simulink model "sampleModel1937"  (R2023a)
settings: Solver=VariableStepAuto  StartTime=0.0  StopTime=10.0  RelTol=1e-3
libraries: hdlsllib x6, simulink x2
settings Model: Creator=user1  LastModifiedBy=user1

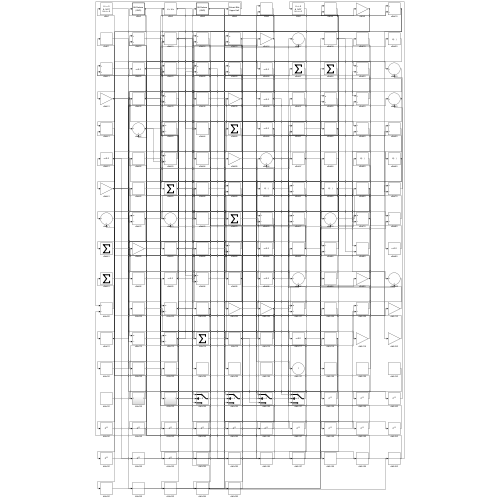
[thumbnail: Simulink's stored preview of the top-level diagram]
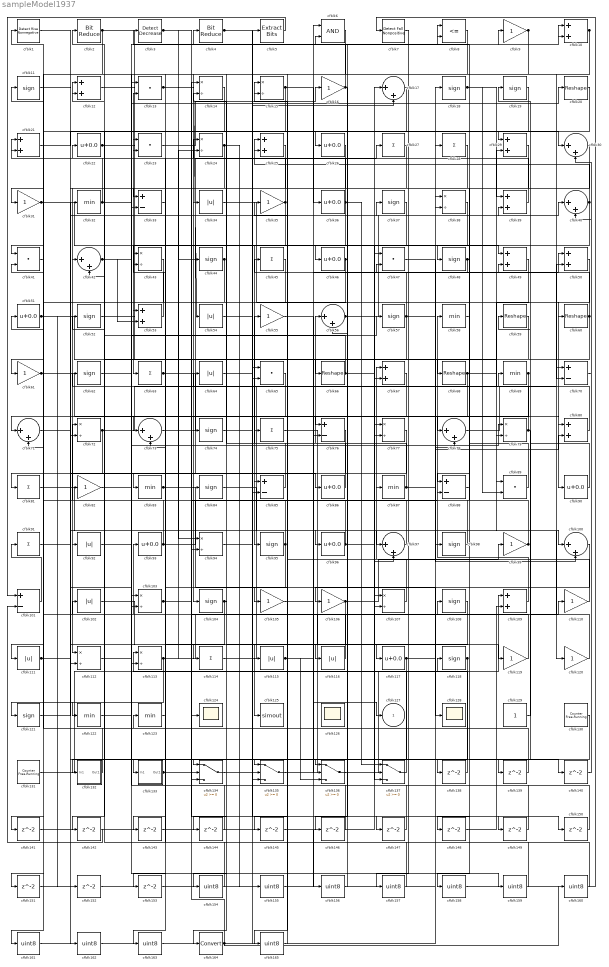
== system sampleModel1937 ==
  cfblk1 : hdlsllib/Logic and Bit Operations/Detect Rise Nonnegative  vinit=0  OutDataTypeStr=boolean
  cfblk{10,12,21,25,29,39,49..50,53,67,80,109} (12 alike) : Sum
  cfblk{17,30,40,42,56,71,73,78,97,100} (10 alike) : Sum  Inputs=|++
  cfblk{33,70,76,85,88,101} (6 alike) : Sum  Inputs=+-
  cfblk{34,54,64,92,102,111,115..116} (8 alike) : Abs  SaturateOnIntegerOverflow=off
  cfblk{14..15,24,38,43,72,77,79,94,103,107,112..113} (13 alike) : Product  Inputs=*/  RndMeth=Zero  SaturateOnIntegerOverflow=on
  cfblk{11,18..19,37,44,48,52,57,62,74,84,95,98,104,108,118,121} (17 alike) : Signum
  cfblk{9,16,31,35,55,61,82,99,105..106,110,119..120} (13 alike) : Gain
  cfblk{27..28,45,63,75,81,91,114} (8 alike) : Sum  Inputs=+
  cfblk{22,26,36,46,51,86,90,93,96,117} (10 alike) : Bias  Bias=0.0  SaturateOnIntegerOverflow=off
  cfblk{32,58,69,83,87,122..123} (7 alike) : MinMax
  cfblk124 : Scope
  cfblk125 : ToWorkspace  VariableName=simout  SaveFormat=Timeseries  SampleTime=-1
  cfblk126 : Scope
      settings: Floating=on
  cfblk128 : Scope
  cfblk129 : Constant  SampleTime=-1
  cfblk{13,23,41,47,65,89} (6 alike) : DotProduct  OutDataTypeStr=Inherit: Inherit via internal rule
  cfblk130 : hdlsllib/Sources/Counter Free-Running  NumBits=16  tsamp=-1
  cfblk131 : hdlsllib/Sources/Counter Free-Running  NumBits=16  tsamp=-1
  cfblk132 : Subsystem
      settings: LibrarySourceBlock=|
      | hdlsllib/Ports &
      | Subsystems/Subsystem
  cfblk133 : Subsystem
      settings: LibrarySourceBlock=|
      | hdlsllib/Ports &
      | Subsystems/Subsystem
  cfblk{134..137} (4 alike) : Switch  SaturateOnIntegerOverflow=off  InputSameDT=off
  cfblk{138..153} (16 alike) : Delay  SampleTime=1
  cfblk{154..163,165} (11 alike) : DataTypeConversion  OutDataTypeStr=uint8  SaturateOnIntegerOverflow=off  RndMeth=Floor
  cfblk164 : DataTypeConversion  SaturateOnIntegerOverflow=off  RndMeth=Floor
  cfblk2 : hdlsllib/Logic and Bit Operations/Bit Reduce  mode=AND
  cfblk{20,59..60,66,68} (5 alike) : Reshape
  cfblk3 : simulink/Logic and Bit Operations/Detect Decrease  vinit=0.0  OutDataTypeStr=boolean
      settings: LibrarySourceBlock=|
      | hdlsllib/Logic and Bit
      | Operations/Detect
      | Decrease
  cfblk4 : hdlsllib/Logic and Bit Operations/Bit Reduce  mode=AND
  cfblk5 : simulink/Logic and Bit Operations/Extract Bits  bitsToExtract=Upper half  numBits=8  bitIdxRange=[0 7]  outScalingMode=Preserve fixed-point scaling
      settings: LibrarySourceBlock=|
      | hdlsllib/Logic and Bit
      | Operations/Extract Bits
  cfblk6 : Logic  AllPortsSameDT=off  OutDataTypeStr=boolean
  cfblk7 : hdlsllib/Logic and Bit Operations/Detect Fall Nonpositive  vinit=0  OutDataTypeStr=boolean
  cfblk8 : RelationalOperator  Operator=<=  OutDataTypeStr=boolean  InputSameDT=off
  cfblk127 : Outport  VectorParamsAs1DForOutWhenUnconnected=off
  wires:
  cfblk108/1 -> cfblk125/1
  cfblk8/1 -> cfblk104/1
  cfblk35/1 -> cfblk93/1, cfblk14/2
  cfblk75/1 -> cfblk117/1
  cfblk109/1 -> cfblk58/1
  cfblk57/1 -> cfblk25/1, cfblk100/2, cfblk137/2
  cfblk68/1 -> cfblk71/1, cfblk100/1
  cfblk29/1 -> cfblk78/1
  cfblk120/1 -> cfblk29/1
  cfblk100/1 -> cfblk106/1
  cfblk56/1 -> cfblk40/1, cfblk97/2
  cfblk40/1 -> cfblk63/1, cfblk25/2
  cfblk50/1 -> cfblk90/1
  cfblk136/1 -> cfblk109/1
  cfblk81/1 -> cfblk96/1
  cfblk2/1 -> cfblk26/1, cfblk31/1
  cfblk12/1 -> cfblk49/1
  cfblk79/1 -> cfblk62/1, cfblk139/1
  cfblk15/1 -> cfblk36/1, cfblk42/2
  cfblk119/1 -> cfblk21/1
  cfblk87/1 -> cfblk56/1, cfblk24/1, cfblk80/2
  cfblk89/1 -> cfblk4/1
  cfblk27/1 -> cfblk112/1
  cfblk131/1 -> cfblk118/1
  cfblk113/1 -> cfblk70/1, cfblk24/2, cfblk151/1
  cfblk114/1 -> cfblk69/1
  cfblk22/1 -> cfblk89/1, cfblk67/2
  cfblk10/1 -> cfblk61/1, cfblk70/2, cfblk145/1
  cfblk62/1 -> cfblk20/1
  cfblk103/1 -> cfblk124/1, cfblk88/2
  cfblk25/1 -> cfblk42/1
  cfblk60/1 -> cfblk15/1, cfblk66/1, cfblk136/2
  cfblk38/1 -> cfblk95/1
  cfblk4/1 -> cfblk107/2, cfblk140/1
  cfblk97/1 -> cfblk67/1
  cfblk47/1 -> cfblk98/1
  cfblk19/1 -> cfblk132/1(In1)
  cfblk34/1 -> cfblk60/1
  cfblk39/1 -> cfblk11/1
  cfblk77/1 -> cfblk92/1
  cfblk66/1 -> cfblk17/1, cfblk12/2
  cfblk99/1 -> cfblk72/1, cfblk8/2
  cfblk85/1 -> cfblk55/1
  cfblk59/1 -> cfblk122/1
  cfblk73/1 -> cfblk27/1
  cfblk110/1 -> cfblk87/1
  cfblk51/1 -> cfblk68/1, cfblk152/1
  cfblk63/1 -> cfblk86/1, cfblk97/1
  cfblk44/1 -> cfblk53/1, cfblk73/2
  cfblk31/1 -> cfblk48/1, cfblk111/1, cfblk94/2
  cfblk23/1 -> cfblk16/1
  cfblk105/1 -> cfblk50/1
  cfblk106/1 -> cfblk134/1, cfblk99/1
  cfblk118/1 -> cfblk137/3, cfblk165/1
  cfblk67/1 -> cfblk74/1
  cfblk24/1 -> cfblk73/1, cfblk155/1
  cfblk83/1 -> cfblk128/1, cfblk115/1
  cfblk55/1 -> cfblk127/1
  cfblk101/1 -> cfblk91/1
  cfblk133/1(Out1) -> cfblk108/1, cfblk147/1
  cfblk88/1 -> cfblk8/1
  cfblk76/1 -> cfblk112/2
  cfblk14/1 -> cfblk41/1
  cfblk21/1 -> cfblk30/1
  cfblk137/1 -> cfblk113/1
  cfblk94/1 -> cfblk17/2
  cfblk102/1 -> cfblk134/2
  cfblk70/1 -> cfblk30/2
  cfblk135/1 -> cfblk110/1
  cfblk45/1 -> cfblk164/1
  cfblk32/1 -> cfblk21/2, cfblk114/1, cfblk119/1
  cfblk26/1 -> cfblk83/1
  cfblk18/1 -> cfblk39/1, cfblk89/2
  cfblk86/1 -> cfblk64/1
  cfblk36/1 -> cfblk135/1, cfblk23/2, cfblk137/1
  cfblk91/1 -> cfblk116/1
  cfblk78/1 -> cfblk50/2
  cfblk53/1 -> cfblk13/2
  cfblk122/1 -> cfblk57/1
  cfblk43/1 -> cfblk113/2
  cfblk54/1 -> cfblk10/1
  cfblk129/1 -> cfblk59/1
  cfblk30/1 -> cfblk72/2
  cfblk84/1 -> cfblk120/1
  cfblk90/1 -> cfblk19/1
  cfblk111/1 -> cfblk37/1, cfblk71/2
  cfblk96/1 -> cfblk52/1, cfblk49/2
  cfblk115/1 -> cfblk9/1, cfblk136/3
  cfblk112/1 -> cfblk79/1
  cfblk116/1 -> cfblk43/1
  cfblk5/1 -> cfblk101/1
  cfblk104/1 -> cfblk143/1, cfblk144/1
  cfblk95/1 -> cfblk51/1, cfblk153/1
  cfblk13/1 -> cfblk54/1, cfblk94/1, cfblk85/2
  cfblk71/1 -> cfblk32/1
  cfblk46/1 -> cfblk76/1, cfblk141/1
  cfblk72/1 -> cfblk29/2, cfblk81/1
  cfblk3/1 -> cfblk75/1, cfblk44/1
  cfblk52/1 -> cfblk76/2
  cfblk20/1 -> cfblk84/1
  cfblk37/1 -> cfblk77/2
  cfblk117/1 -> cfblk78/2, cfblk142/1
  cfblk64/1 -> cfblk5/1
  cfblk69/1 -> cfblk136/1, cfblk105/1
  cfblk28/1 -> cfblk34/1
  cfblk107/1 -> cfblk35/1
  cfblk132/1(Out1) -> cfblk41/2
  cfblk80/1 -> cfblk12/1
  cfblk93/1 -> cfblk47/1, cfblk2/1
  cfblk33/1 -> cfblk133/1(In1)
  cfblk42/1 -> cfblk10/2, cfblk53/2
  cfblk98/1 -> cfblk23/1
  cfblk121/1 -> cfblk39/2
  cfblk48/1 -> cfblk88/1, cfblk47/2
  cfblk41/1 -> cfblk121/1
  cfblk92/1 -> cfblk134/3
  cfblk61/1 -> cfblk80/1, cfblk103/2, cfblk85/1
  cfblk16/1 -> cfblk46/1, cfblk3/1
  cfblk9/1 -> cfblk33/1, cfblk33/2
  cfblk49/1 -> cfblk79/2
  cfblk11/1 -> cfblk138/1
  cfblk138/1 -> cfblk56/2
  cfblk139/1 -> cfblk1/1
  cfblk140/1 -> cfblk40/2
  cfblk141/1 -> cfblk107/1
  cfblk142/1 -> cfblk101/2
  cfblk143/1 -> cfblk43/2
  cfblk144/1 -> cfblk103/1
  cfblk17/1 -> cfblk146/1
  cfblk146/1 -> cfblk13/1
  cfblk147/1 -> cfblk135/2
  cfblk58/1 -> cfblk148/1
  cfblk148/1 -> cfblk109/2
  cfblk134/1 -> cfblk149/1
  cfblk149/1 -> cfblk77/1
  cfblk74/1 -> cfblk150/1
  cfblk150/1 -> cfblk15/2
  cfblk151/1 -> cfblk135/3
  cfblk152/1 -> cfblk38/1
  cfblk153/1 -> cfblk38/2
  cfblk6/1 -> cfblk154/1
  cfblk154/1 -> cfblk22/1
  cfblk155/1 -> cfblk6/1
  cfblk145/1 -> cfblk156/1
  cfblk156/1 -> cfblk6/2
  cfblk7/1 -> cfblk157/1
  cfblk157/1 -> cfblk102/1
  cfblk130/1 -> cfblk158/1
  cfblk158/1 -> cfblk7/1
  cfblk82/1 -> cfblk159/1
  cfblk159/1 -> cfblk123/1
  cfblk160/1 -> cfblk82/1
  cfblk65/1 -> cfblk161/1
  cfblk161/1 -> cfblk28/1
  cfblk1/1 -> cfblk162/1
  cfblk162/1 -> cfblk65/1
  cfblk123/1 -> cfblk163/1
  cfblk163/1 -> cfblk65/2
  cfblk164/1 -> cfblk160/1, cfblk14/1, cfblk18/1
  cfblk165/1 -> cfblk45/1

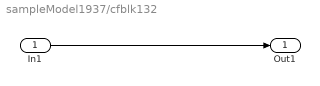
== system sampleModel1937/cfblk132 ==
  In1 : Inport
  Out1 : Outport
  wires:
  In1/1 -> Out1/1

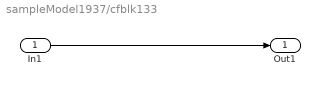
== system sampleModel1937/cfblk133 ==
  In1 : Inport
  Out1 : Outport
  wires:
  In1/1 -> Out1/1
